simulink model "Problem4"  (R2020b)
settings: Solver=VariableStepAuto  StartTime=0.0  StopTime=10.0  RelTol=1e-3
settings Model: Creator=amolg  LastModifiedBy=amolg

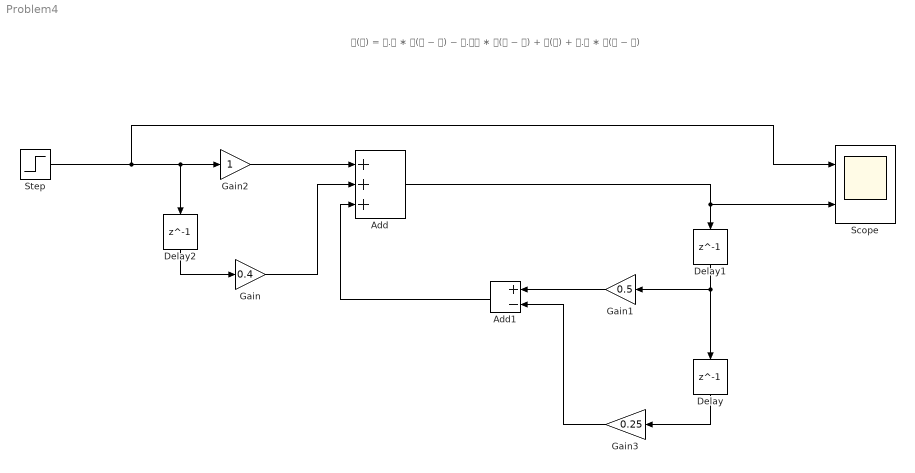
== system Problem4 ==
  note: 𝐲(𝐧) = 𝟎.𝟓 ∗ 𝐲(𝐧 − 𝟏) − 𝟎.𝟐𝟓 ∗ 𝐲(𝐧 − 𝟐) + 𝐱(𝐧) + 𝟎.𝟒 ∗ 𝐱(𝐧 − 𝟏)
  Add : Sum  Inputs=+++
  Add1 : Sum  Inputs=+-
  Delay : Delay  DelayLength=1
  Delay1 : Delay  DelayLength=1
  Delay2 : Delay  DelayLength=1
  Gain : Gain  Gain=0.4
  Gain1 : Gain  Gain=0.5
  Gain2 : Gain
  Gain3 : Gain  Gain=0.25
  Scope : Scope  NumInputPorts=2
  Step : Step  SampleTime=0
  wires:
  Gain2/1 -> Add/1
  Delay2/1 -> Gain/1
  Gain/1 -> Add/2
  Add/1 -> Delay1/1, Scope/2
  Delay1/1 -> Delay/1, Gain1/1
  Gain1/1 -> Add1/1
  Delay/1 -> Gain3/1
  Gain3/1 -> Add1/2
  Add1/1 -> Add/3
  Step/1 -> Scope/1, Delay2/1, Gain2/1
